simulink model "Unipolar_Carrier_Signal_Based_SVPWM"  (R2023a)
settings: Solver=VariableStepAuto  StartTime=0.0  StopTime=2  MaxStep=1e-5  RelTol=1e-3
libraries: spsMosfetLib x12, spsDiodeLib x6, simulink x4, spsVoltageMeasurementLib x4, spsDCVoltageSourceLib x2, spsGroundLib x2, spsSeriesRLCBranchLib x2, spsAsynchronousMachineSIUnitsLib x1, spsCurrentMeasurementLib x1, spsStairGeneratorLib x1, spsThreePhaseVIMeasurementLib x1, spspowerguiLib x1
settings Model: Creator=Vigneshwaran R  LastModifiedBy=Vigneshwaran R
settings DataIOCC: SaveOutput=off  SaveState=on  SignalLogging=off  DSMLogging=off  ReturnWorkspaceOutputs=off  LoggingToFile=on
settings ModelReferenceCC: EnableRefExpFcnMdlSchedulingChecks=on

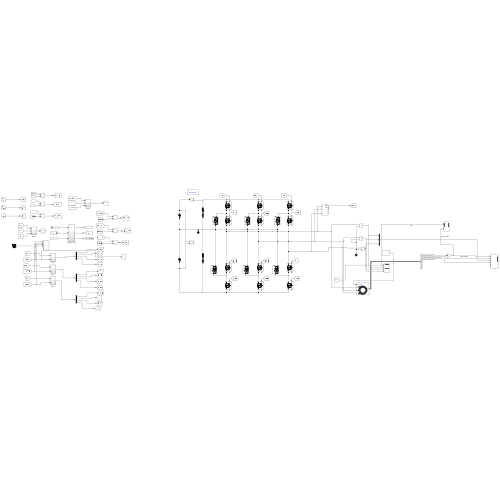
[thumbnail: Simulink's stored preview of the top-level diagram]
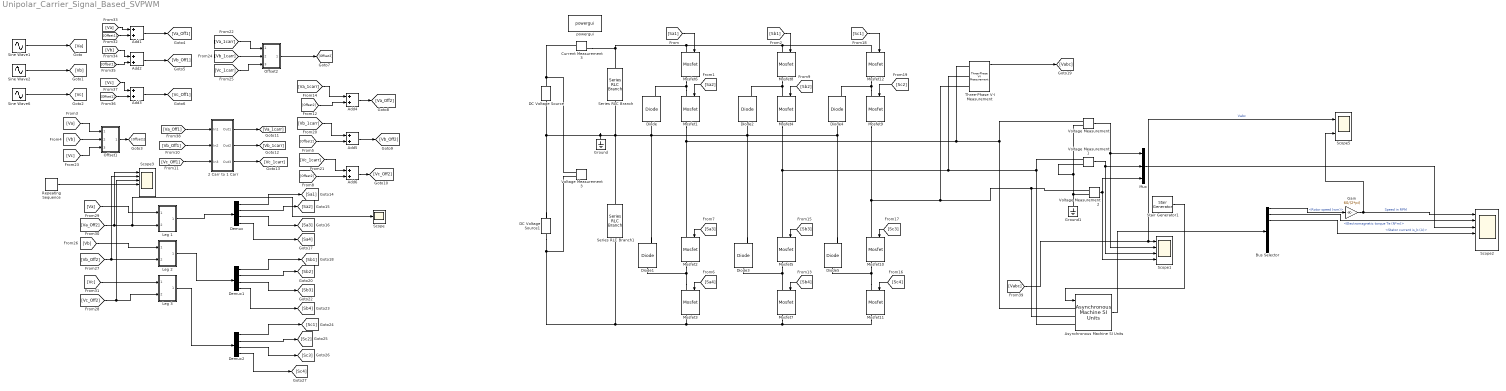
== system Unipolar_Carrier_Signal_Based_SVPWM ==
  2 Carr to 1 Carr : Subsystem
  Add{1..6} (6 alike) : Sum
  Asynchronous Machine SI Units : spsAsynchronousMachineSIUnitsLib/Asynchronous Machine SI Units  RotorType=Squirrel-cage  PresetModel="15:  5.4 HP (4KW)   400 V  50Hz 1430 RPM"  MechanicalLoad=Torque Tm  ShowDetailedParameters=on  ReferenceFrame=Rotor  Units=SI  MeasurementBus=off  NominalParameters=[4000 400 50]  VoltageRatio=1  Stator=[1.405 0.005839]  Rotor=[1.395 0.005839]  Cage1=[0.4155 0.002066]  Cage2=[0.4168 0.0003495]  Lm=0.1722  Mechanical=[0.0131 0.002985 2]  PolePairs=2  InitialConditions=[0 0 0 0 0 0 0 0]  SimulateSaturation=off  Saturation=[14.03593122, 27.81365428, 53.79336849, 72.68890987, 97.98006896, 148.6815601, 215.7428561, 302.9841135, 428.7778367 ; 230, 322, 414, 460, 506, 552, 598, 644, 690]  LoadFlowParameters=1492000  TsPowergui=0  TsBlock=-1  IterativeModel=Trapezoidal non iterative  IterativeDiscreteModel=Trapezoidal non iterative  Pmec=1.492e+006
  Bus Selector : BusSelector  OutputSignals=Mechanical.Rotor speed (wm),Mechanical.Electromagnetic torque Te (N*m),Stator measurements.Stator current is_b (A),Stator measurements.Stator flux phis_d (V s),Stator measurements.Stator flux phis_q (V s),Stator measurements.Stator current is_a (A),Stator measurements.Stator current is_b (A),Stator measurements.Stator current is_c (A)
  Current Measurement3 : spsCurrentMeasurementLib/Current Measurement  PhasorSimulation=off  OutputType=Complex  PSBequivalent=0
  DC Voltage Source : spsDCVoltageSourceLib/DC Voltage Source  Amplitude=380  Measurements=None
  DC Voltage Source1 : spsDCVoltageSourceLib/DC Voltage Source  Amplitude=380  Measurements=None
  Demux : Demux
  Demux1 : Demux
  Demux2 : Demux
  Diode{,1..5} (6 alike) : spsDiodeLib/Diode  Ron=0.001  Lon=0  Vf=0.8  IC=0  UseSnubber=0  Rs=500  Cs=250e-9  Measurements=on
  Gain : Gain  Gain=60/(2*pi)
  Ground : spsGroundLib/Ground  LConnTagsString=a
  Ground1 : spsGroundLib/Ground  LConnTagsString=a
  Leg 1 : Subsystem
  Leg 2 : Subsystem
  Leg 3 : Subsystem
  Mosfet{1..12} (12 alike) : spsMosfetLib/Mosfet  Ron=0.1  Lon=0  Rd=0.01  Vfd=0  IC=0  Rs=1e5  Cs=inf  Measurements=on
  Mux : Mux  Inputs=3
  Offset1 : Subsystem
  Offset2 : Subsystem
  Repeating Sequence : simulink/Sources/Repeating Sequence  rep_seq_t=[0 2.5e-5 5e-5 7.5e-5 10e-5]  rep_seq_y=[0.5 1 0.5 0 0.5 ]
  Scope : Scope
  Scope1 : Scope  NumInputPorts=4
  Scope2 : Scope  NumInputPorts=6
  Scope3 : Scope  NumInputPorts=6
  Scope5 : Scope  NumInputPorts=2
  Series RLC Branch : spsSeriesRLCBranchLib/Series RLC Branch  LConnTagsString=__new0  RConnTagsString=__new0  BranchType=RC  Resistance=0.1  Inductance=1e-3  SetiL0=off  InitialCurrent=0  Capacitance=4.7e-3  Setx0=off  InitialVoltage=0  Measurements=None
  Series RLC Branch1 : spsSeriesRLCBranchLib/Series RLC Branch  LConnTagsString=__new0  RConnTagsString=__new0  BranchType=RC  Resistance=0.1  Inductance=1e-3  SetiL0=off  InitialCurrent=0  Capacitance=4.7e-3  Setx0=off  InitialVoltage=0  Measurements=None
  Sine Wave1 : Sin  Frequency=2*pi*50  SampleTime=0
  Sine Wave2 : Sin  Frequency=2*pi*50  Phase=2*pi/3  SampleTime=0
  Sine Wave6 : Sin  Frequency=2*pi*50  Phase=4*pi/3  SampleTime=0
  Stair Generator1 : spsStairGeneratorLib/Stair Generator  t=[0 1]  e=[0 10]  Ts=0
  Three-Phase V-I Measurement : spsThreePhaseVIMeasurementLib/Three-Phase V-I Measurement  VoltageMeasurement=phase-to-phase  SetLabelV=off  LabelV=Vabc  Vpu=off  VpuLL=off  CurrentMeasurement=yes  SetLabelI=off  LabelI=Iabc  Ipu=off  Pbase=100e6  Vbase=500e3  OutputType=Complex  PhasorSimulation=off  PSBequivalent=0
  Voltage Measurement{,1..3} (4 alike) : spsVoltageMeasurementLib/Voltage Measurement  PhasorSimulation=off  OutputType=Complex  PSBequivalent=0
  powergui : spspowerguiLib/powergui  Priority=1  SimulationMode=Continuous  SampleTime=50e-6  frequency=60  Iterations=50  frequencyindice=50  Pbase=100e6  ErrMax=1e-4  UnitsV=kV  UnitsW=MW  buscounter=0  FunctionMessages=off  echomessages=off  EnableUseOfTLC=off  CurrentSourceSwitches=off  DisableSnubberDevices=off  DisableRonSwitches=off  DisableVfSwitches=off  DisplayEquations=off  AutomaticDiscreteSolvers=off  SolverType=Tustin/Backward Euler (TBE)  Interpol=off  ExternalGateDelay=off  methode=off  Ts=100  x0status=blocks  SPID=on  SwTol=0  HookPort=off  NonlinearTolerance=1e-4  nMaxIteration=100  ContinueOnMaxIteration=off  RestoreLinks=warning  ResistiveCurrentMeasurement=off  Frange=[0:2:500]  Ylog=off  Xlog=on  ShowGrid=off  save=off  variable=ZData  structure=0  ZoomFFT=off  StartTime=0.0  cycles=1  DisplayStyle=1  fundamental=60  FreqAxis=off  MaxFrequency=1000  frequencyindicesteady=1  RmsSteady=1  display=off
  wires:
  [Sa2] -> Mosfet1/1
  [Sa4] -> Mosfet3/1
  [Sa3] -> Mosfet2/1
  [Sa1] -> Mosfet6/1
  [Sb1] -> Mosfet8/1
  [Sb3] -> Mosfet5/1
  [Sb4] -> Mosfet7/1
  [Sb2] -> Mosfet4/1
  [Sc2] -> Mosfet9/1
  [Sc4] -> Mosfet11/1
  [Sc3] -> Mosfet10/1
  [Sc1] -> Mosfet12/1
  Three-Phase V-I Measurement/1 -> [Vabc]
  [Offset2] -> Add4/2
  [Va_1carr] -> Offset2/1(In1)
  [Offset2] -> Add5/2
  [Offset2] -> Add6/2
  [Vc] -> Leg 3/1(In1)
  [Va_1carr] -> Add4/1
  [Vb_1carr] -> Add5/1
  [Vb] -> Leg 2/1(In1)
  [Va] -> Leg 1/1(In1)
  [Vc_Off2] -> Leg 3/2(In2), Scope3/3
  Add6/1 -> [Vc_Off2]
  Add4/1 -> [Va_Off2]
  2 Carr to 1 Carr/3(Out3) -> [Vc_1carr]
  Offset2/1(Out1) -> [Offset2]
  [Vc_Off1] -> 2 Carr to 1 Carr/3(In3)
  2 Carr to 1 Carr/1(Out1) -> [Va_1carr]
  Offset1/1(Out1) -> [Offset1]
  [Vc_1carr] -> Offset2/3(In3)
  Add1/1 -> [Va_Off1]
  [Va] -> Offset1/1(In1)
  [Vc] -> Offset1/3(In3)
  [Vb] -> Offset1/2(In2)
  [Va_Off2] -> Scope3/1, Scope/1, Leg 1/2(In2)
  [Offset1] -> Add2/2
  [Vb] -> Add2/1
  Add5/1 -> [Vb_Off2]
  [Vb_Off1] -> 2 Carr to 1 Carr/2(In2)
  [Vb_1carr] -> Offset2/2(In2)
  [Offset1] -> Add3/2
  [Vb_Off2] -> Scope3/2, Leg 2/2(In2)
  [Va] -> Add1/1
  [Offset1] -> Add1/2
  [Vc] -> Add3/1
  [Vc_1carr] -> Add6/1
  2 Carr to 1 Carr/2(Out2) -> [Vb_1carr]
  [Va_Off1] -> 2 Carr to 1 Carr/1(In1)
  Add2/1 -> [Vb_Off1]
  Add3/1 -> [Vc_Off1]
  Leg 1/1(Out1) -> Demux/1
  Demux/1 -> [Sa1]
  Demux/2 -> [Sa2]
  Demux/3 -> [Sa3]
  Demux/4 -> [Sa4]
  Demux1/4 -> [Sb4]
  Demux1/3 -> [Sb3]
  Demux1/2 -> [Sb2]
  Demux1/1 -> [Sb1]
  Leg 2/1(Out1) -> Demux1/1
  Leg 3/1(Out1) -> Demux2/1
  Demux2/1 -> [Sc1]
  Demux2/2 -> [Sc2]
  Demux2/3 -> [Sc3]
  Demux2/4 -> [Sc4]
  Voltage Measurement/1 -> Mux/1, Scope1/2
  Voltage Measurement1/1 -> Scope1/3, Mux/2
  Voltage Measurement2/1 -> Scope1/4, Mux/3
  Mux/1 -> Scope2/3
  Asynchronous Machine SI Units/1 -> Bus Selector/1
  Bus Selector/1 -> Gain/1  "<Rotor speed (wm)>"
  Bus Selector/2 -> Scope2/2  "<Electromagnetic torque Te (N*m)>"
  Stair Generator1/1 -> Asynchronous Machine SI Units/1
  Repeating Sequence/1 -> Scope3/4
  Gain/1 -> Scope2/1, Scope5/2  "Speed in RPM"
  [Vabc] -> Scope5/1, Scope1/1  "Vabc"
  Bus Selector/3 -> Scope2/4  "<Stator current is_b (A)>"
  Sine Wave2/1 -> [Vb]
  Sine Wave1/1 -> [Va]
  Sine Wave6/1 -> [Vc]
  connections:
  Diode4/LConn1 -- Series RLC Branch1/LConn1 -- Series RLC Branch/RConn1 -- Ground/LConn1 -- DC Voltage Source/LConn1 -- DC Voltage Source1/RConn1 -- Diode1/RConn1 -- Diode/LConn1 -- Diode2/LConn1 -- Diode3/RConn1 -- Diode5/RConn1
  Series RLC Branch/LConn1 -- Current Measurement3/RConn1 -- Mosfet8/LConn1 -- Mosfet12/LConn1 -- Mosfet6/LConn1
  Mosfet3/LConn1 -- Mosfet2/RConn1 -- Diode1/LConn1
  Three-Phase V-I Measurement/LConn1 -- Mosfet1/RConn1 -- Mosfet2/LConn1 -- Asynchronous Machine SI Units/LConn1 -- Voltage Measurement/LConn1
  Mosfet1/LConn1 -- Mosfet6/RConn1 -- Diode/RConn1
  Voltage Measurement3/LConn2 -- DC Voltage Source1/LConn1 -- Series RLC Branch1/RConn1 -- Mosfet7/RConn1 -- Mosfet11/RConn1 -- Mosfet3/RConn1
  Mosfet5/RConn1 -- Mosfet7/LConn1 -- Diode3/LConn1
  Mosfet8/RConn1 -- Mosfet4/LConn1 -- Diode2/RConn1
  Mosfet11/LConn1 -- Mosfet10/RConn1 -- Diode5/LConn1
  Mosfet9/LConn1 -- Mosfet12/RConn1 -- Diode4/RConn1
  Mosfet4/RConn1 -- Asynchronous Machine SI Units/LConn3 -- Voltage Measurement1/LConn1 -- Three-Phase V-I Measurement/LConn2 -- Mosfet5/LConn1
  Mosfet9/RConn1 -- Asynchronous Machine SI Units/LConn2 -- Voltage Measurement2/LConn1 -- Three-Phase V-I Measurement/LConn3 -- Mosfet10/LConn1
  Current Measurement3/LConn1 -- Voltage Measurement3/LConn1 -- DC Voltage Source/RConn1
  Voltage Measurement/LConn2 -- Ground1/LConn1 -- Voltage Measurement2/LConn2 -- Voltage Measurement1/LConn2

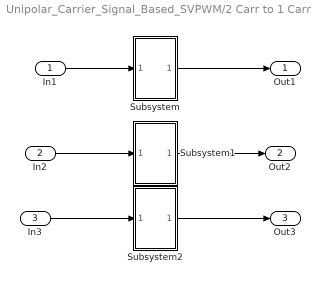
== system Unipolar_Carrier_Signal_Based_SVPWM/2 Carr to 1 Carr ==
  In1 : Inport
  In2 : Inport  Port=2
  In3 : Inport  Port=3
  Subsystem : Subsystem
  Subsystem1 : Subsystem
  Subsystem2 : Subsystem
  Out1 : Outport
  Out2 : Outport  Port=2
  Out3 : Outport  Port=3
  wires:
  In2/1 -> Subsystem1/1(In1)
  In3/1 -> Subsystem2/1(In1)
  Subsystem1/1(Out1) -> Out2/1
  Subsystem2/1(Out1) -> Out3/1
  Subsystem/1(Out1) -> Out1/1
  In1/1 -> Subsystem/1(In1)

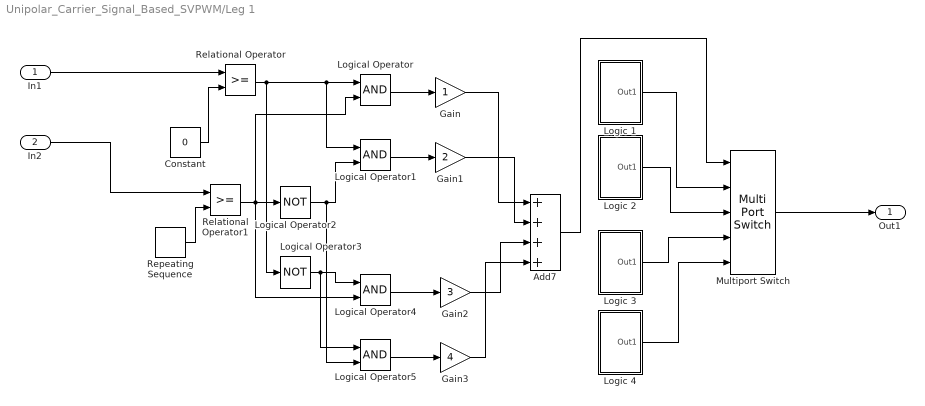
== system Unipolar_Carrier_Signal_Based_SVPWM/Leg 1 ==
  In1 : Inport
  In2 : Inport  Port=2
  Add7 : Sum  Inputs=++++
  Constant : Constant  Value=0
  Gain : Gain
  Gain1 : Gain  Gain=2
  Gain2 : Gain  Gain=3
  Gain3 : Gain  Gain=4
  Logic 1 : Subsystem
  Logic 2 : Subsystem
  Logic 3 : Subsystem
  Logic 4 : Subsystem
  Logical Operator{,1,4..5} (4 alike) : Logic  AllPortsSameDT=off  OutDataTypeStr=boolean
  Logical Operator2 : Logic  Operator=NOT  AllPortsSameDT=off  OutDataTypeStr=boolean
  Logical Operator3 : Logic  Operator=NOT  AllPortsSameDT=off  OutDataTypeStr=boolean
  Multiport Switch : MultiPortSwitch  Inputs=4  SaturateOnIntegerOverflow=off  InputSameDT=off
  Relational Operator : RelationalOperator  OutDataTypeStr=boolean  RndMeth=Simplest  InputSameDT=off
  Relational Operator1 : RelationalOperator  OutDataTypeStr=boolean  RndMeth=Simplest  InputSameDT=off
  Repeating Sequence : simulink/Sources/Repeating Sequence  rep_seq_t=[0 2.5e-5 5e-5 7.5e-5 10e-5]  rep_seq_y=[0.5 1 0.5 0 0.5 ]
  Out1 : Outport
  wires:
  Logical Operator5/1 -> Gain3/1
  Logical Operator1/1 -> Gain1/1
  Constant/1 -> Relational Operator/2
  Logical Operator3/1 -> Logical Operator5/1, Logical Operator4/1
  Logic 4/1(Out1) -> Multiport Switch/5
  Logical Operator4/1 -> Gain2/1
  Logical Operator2/1 -> Logical Operator5/2, Logical Operator1/2
  Relational Operator1/1 -> Logical Operator4/2, Logical Operator2/1, Logical Operator/2
  Gain2/1 -> Add7/3
  In2/1 -> Relational Operator1/1
  Add7/1 -> Multiport Switch/1
  Repeating Sequence/1 -> Relational Operator1/2
  Relational Operator/1 -> Logical Operator3/1, Logical Operator1/1, Logical Operator/1
  Logic 3/1(Out1) -> Multiport Switch/4
  Gain/1 -> Add7/1
  Gain1/1 -> Add7/2
  Logic 2/1(Out1) -> Multiport Switch/3
  Logic 1/1(Out1) -> Multiport Switch/2
  Gain3/1 -> Add7/4
  Logical Operator/1 -> Gain/1
  Multiport Switch/1 -> Out1/1
  In1/1 -> Relational Operator/1

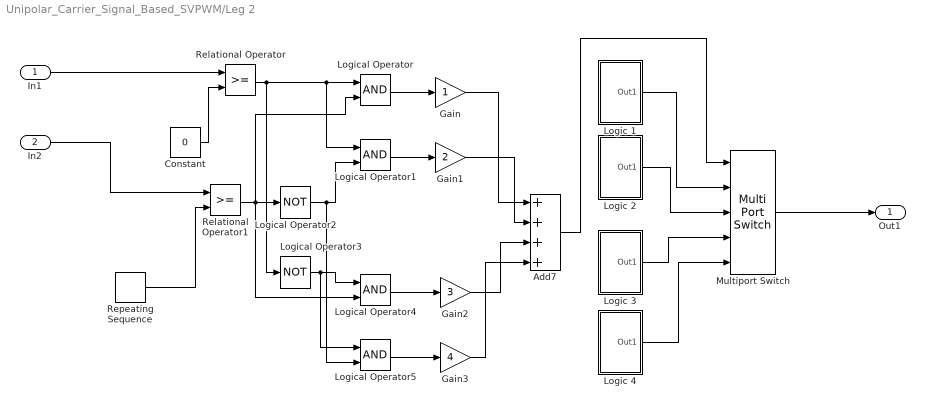
== system Unipolar_Carrier_Signal_Based_SVPWM/Leg 2 ==
  In1 : Inport
  In2 : Inport  Port=2
  Add7 : Sum  Inputs=++++
  Constant : Constant  Value=0
  Gain : Gain
  Gain1 : Gain  Gain=2
  Gain2 : Gain  Gain=3
  Gain3 : Gain  Gain=4
  Logic 1 : Subsystem
  Logic 2 : Subsystem
  Logic 3 : Subsystem
  Logic 4 : Subsystem
  Logical Operator{,1,4..5} (4 alike) : Logic  AllPortsSameDT=off  OutDataTypeStr=boolean
  Logical Operator2 : Logic  Operator=NOT  AllPortsSameDT=off  OutDataTypeStr=boolean
  Logical Operator3 : Logic  Operator=NOT  AllPortsSameDT=off  OutDataTypeStr=boolean
  Multiport Switch : MultiPortSwitch  Inputs=4  SaturateOnIntegerOverflow=off  InputSameDT=off
  Relational Operator : RelationalOperator  OutDataTypeStr=boolean  RndMeth=Simplest  InputSameDT=off
  Relational Operator1 : RelationalOperator  OutDataTypeStr=boolean  RndMeth=Simplest  InputSameDT=off
  Repeating Sequence : simulink/Sources/Repeating Sequence  rep_seq_t=[0 2.5e-5 5e-5 7.5e-5 10e-5]  rep_seq_y=[0.5 1 0.5 0 0.5 ]
  Out1 : Outport
  wires:
  In1/1 -> Relational Operator/1
  Multiport Switch/1 -> Out1/1
  Logical Operator/1 -> Gain/1
  Gain3/1 -> Add7/4
  Logic 1/1(Out1) -> Multiport Switch/2
  Logic 2/1(Out1) -> Multiport Switch/3
  Gain1/1 -> Add7/2
  Gain/1 -> Add7/1
  Logic 3/1(Out1) -> Multiport Switch/4
  Relational Operator/1 -> Logical Operator/1, Logical Operator1/1, Logical Operator3/1
  Repeating Sequence/1 -> Relational Operator1/2
  Add7/1 -> Multiport Switch/1
  In2/1 -> Relational Operator1/1
  Gain2/1 -> Add7/3
  Relational Operator1/1 -> Logical Operator/2, Logical Operator2/1, Logical Operator4/2
  Logical Operator2/1 -> Logical Operator1/2, Logical Operator5/2
  Logical Operator4/1 -> Gain2/1
  Logic 4/1(Out1) -> Multiport Switch/5
  Logical Operator3/1 -> Logical Operator4/1, Logical Operator5/1
  Constant/1 -> Relational Operator/2
  Logical Operator1/1 -> Gain1/1
  Logical Operator5/1 -> Gain3/1

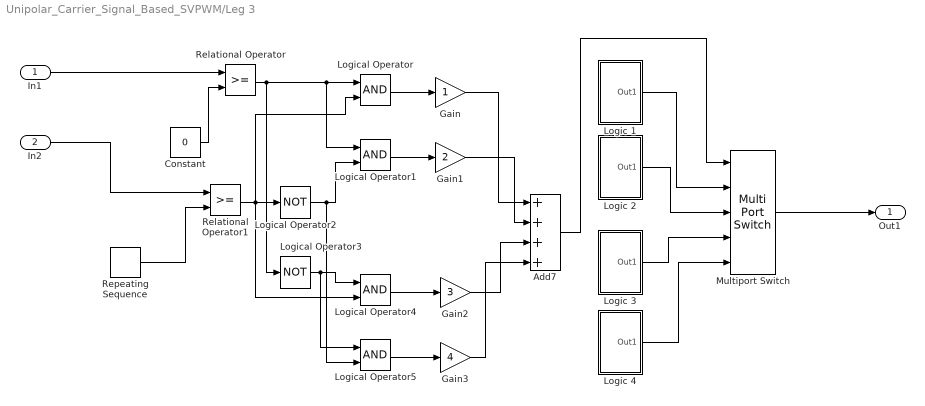
== system Unipolar_Carrier_Signal_Based_SVPWM/Leg 3 ==
  In1 : Inport
  In2 : Inport  Port=2
  Add7 : Sum  Inputs=++++
  Constant : Constant  Value=0
  Gain : Gain
  Gain1 : Gain  Gain=2
  Gain2 : Gain  Gain=3
  Gain3 : Gain  Gain=4
  Logic 1 : Subsystem
  Logic 2 : Subsystem
  Logic 3 : Subsystem
  Logic 4 : Subsystem
  Logical Operator{,1,4..5} (4 alike) : Logic  AllPortsSameDT=off  OutDataTypeStr=boolean
  Logical Operator2 : Logic  Operator=NOT  AllPortsSameDT=off  OutDataTypeStr=boolean
  Logical Operator3 : Logic  Operator=NOT  AllPortsSameDT=off  OutDataTypeStr=boolean
  Multiport Switch : MultiPortSwitch  Inputs=4  SaturateOnIntegerOverflow=off  InputSameDT=off
  Relational Operator : RelationalOperator  OutDataTypeStr=boolean  RndMeth=Simplest  InputSameDT=off
  Relational Operator1 : RelationalOperator  OutDataTypeStr=boolean  RndMeth=Simplest  InputSameDT=off
  Repeating Sequence : simulink/Sources/Repeating Sequence  rep_seq_t=[0 2.5e-5 5e-5 7.5e-5 10e-5]  rep_seq_y=[0.5 1 0.5 0 0.5 ]
  Out1 : Outport
  wires:
  Logical Operator5/1 -> Gain3/1
  Logical Operator1/1 -> Gain1/1
  Constant/1 -> Relational Operator/2
  Logical Operator3/1 -> Logical Operator5/1, Logical Operator4/1
  Logic 4/1(Out1) -> Multiport Switch/5
  Logical Operator4/1 -> Gain2/1
  Logical Operator2/1 -> Logical Operator5/2, Logical Operator1/2
  Relational Operator1/1 -> Logical Operator4/2, Logical Operator2/1, Logical Operator/2
  Gain2/1 -> Add7/3
  In2/1 -> Relational Operator1/1
  Add7/1 -> Multiport Switch/1
  Repeating Sequence/1 -> Relational Operator1/2
  Relational Operator/1 -> Logical Operator3/1, Logical Operator1/1, Logical Operator/1
  Logic 3/1(Out1) -> Multiport Switch/4
  Gain/1 -> Add7/1
  Gain1/1 -> Add7/2
  Logic 2/1(Out1) -> Multiport Switch/3
  Logic 1/1(Out1) -> Multiport Switch/2
  Gain3/1 -> Add7/4
  Logical Operator/1 -> Gain/1
  Multiport Switch/1 -> Out1/1
  In1/1 -> Relational Operator/1

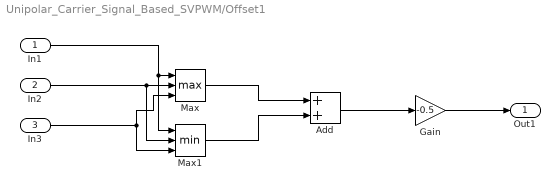
== system Unipolar_Carrier_Signal_Based_SVPWM/Offset1 ==
  In1 : Inport
  In2 : Inport  Port=2
  In3 : Inport  Port=3
  Add : Sum
  Gain : Gain  Gain=-0.5
  Max : MinMax  Function=max  Inputs=3
  Max1 : MinMax  Inputs=3
  Out1 : Outport
  wires:
  In2/1 -> Max1/2, Max/2
  In1/1 -> Max1/1, Max/1
  Max/1 -> Add/1
  In3/1 -> Max/3, Max1/3
  Gain/1 -> Out1/1
  Max1/1 -> Add/2
  Add/1 -> Gain/1

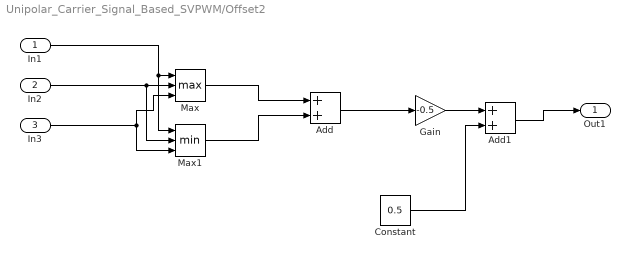
== system Unipolar_Carrier_Signal_Based_SVPWM/Offset2 ==
  In1 : Inport
  In2 : Inport  Port=2
  In3 : Inport  Port=3
  Add : Sum
  Add1 : Sum
  Constant : Constant  Value=0.5
  Gain : Gain  Gain=-0.5
  Max : MinMax  Function=max  Inputs=3
  Max1 : MinMax  Inputs=3
  Out1 : Outport
  wires:
  Add/1 -> Gain/1
  Max1/1 -> Add/2
  In3/1 -> Max1/3, Max/3
  Max/1 -> Add/1
  In1/1 -> Max/1, Max1/1
  In2/1 -> Max/2, Max1/2
  Gain/1 -> Add1/1
  Constant/1 -> Add1/2
  Add1/1 -> Out1/1

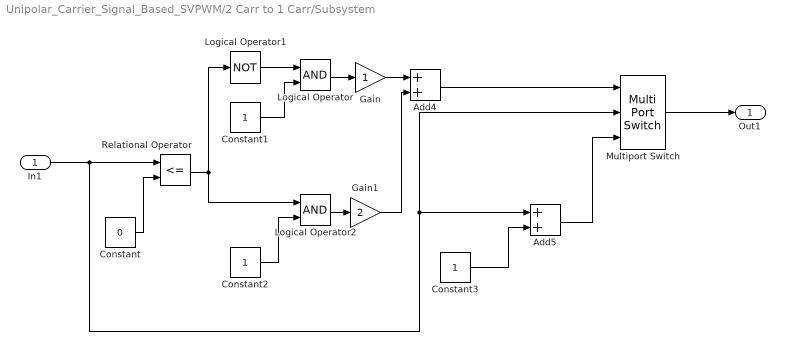
== system Unipolar_Carrier_Signal_Based_SVPWM/2 Carr to 1 Carr/Subsystem ==
  In1 : Inport
  Add4 : Sum
  Add5 : Sum
  Constant : Constant  Value=0
  Constant1 : Constant
  Constant2 : Constant
  Constant3 : Constant
  Gain : Gain
  Gain1 : Gain  Gain=2
  Logical Operator : Logic  AllPortsSameDT=off  OutDataTypeStr=boolean
  Logical Operator1 : Logic  Operator=NOT  AllPortsSameDT=off  OutDataTypeStr=boolean
  Logical Operator2 : Logic  AllPortsSameDT=off  OutDataTypeStr=boolean
  Multiport Switch : MultiPortSwitch  Inputs=2  SaturateOnIntegerOverflow=off  InputSameDT=off
  Relational Operator : RelationalOperator  Operator=<=  OutDataTypeStr=boolean  RndMeth=Simplest  InputSameDT=off
  Out1 : Outport
  wires:
  Gain1/1 -> Add4/2
  In1/1 -> Relational Operator/1, Add5/1, Multiport Switch/2
  Add5/1 -> Multiport Switch/3
  Logical Operator1/1 -> Logical Operator/1
  Logical Operator/1 -> Gain/1
  Constant1/1 -> Logical Operator/2
  Logical Operator2/1 -> Gain1/1
  Multiport Switch/1 -> Out1/1
  Gain/1 -> Add4/1
  Relational Operator/1 -> Logical Operator1/1, Logical Operator2/1
  Constant2/1 -> Logical Operator2/2
  Constant/1 -> Relational Operator/2
  Add4/1 -> Multiport Switch/1
  Constant3/1 -> Add5/2

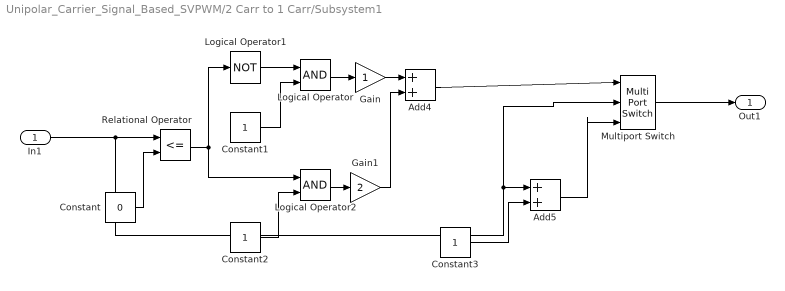
== system Unipolar_Carrier_Signal_Based_SVPWM/2 Carr to 1 Carr/Subsystem1 ==
  In1 : Inport
  Add4 : Sum
  Add5 : Sum
  Constant : Constant  Value=0
  Constant1 : Constant
  Constant2 : Constant
  Constant3 : Constant
  Gain : Gain
  Gain1 : Gain  Gain=2
  Logical Operator : Logic  AllPortsSameDT=off  OutDataTypeStr=boolean
  Logical Operator1 : Logic  Operator=NOT  AllPortsSameDT=off  OutDataTypeStr=boolean
  Logical Operator2 : Logic  AllPortsSameDT=off  OutDataTypeStr=boolean
  Multiport Switch : MultiPortSwitch  Inputs=2  SaturateOnIntegerOverflow=off  InputSameDT=off
  Relational Operator : RelationalOperator  Operator=<=  OutDataTypeStr=boolean  RndMeth=Simplest  InputSameDT=off
  Out1 : Outport
  wires:
  Constant3/1 -> Add5/2
  Add4/1 -> Multiport Switch/1
  Constant/1 -> Relational Operator/2
  Constant2/1 -> Logical Operator2/2
  Relational Operator/1 -> Logical Operator2/1, Logical Operator1/1
  Gain/1 -> Add4/1
  Multiport Switch/1 -> Out1/1
  Logical Operator2/1 -> Gain1/1
  Constant1/1 -> Logical Operator/2
  Logical Operator/1 -> Gain/1
  Logical Operator1/1 -> Logical Operator/1
  Add5/1 -> Multiport Switch/3
  In1/1 -> Relational Operator/1, Add5/1, Multiport Switch/2
  Gain1/1 -> Add4/2

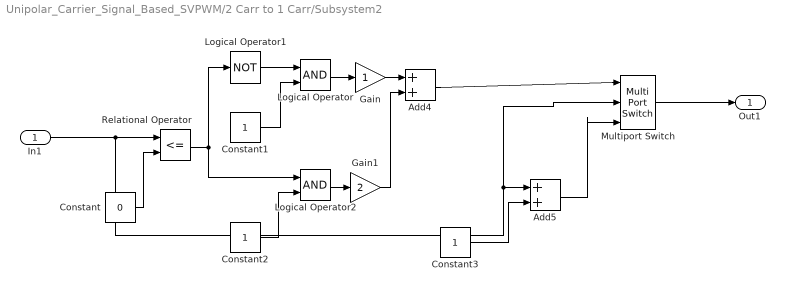
== system Unipolar_Carrier_Signal_Based_SVPWM/2 Carr to 1 Carr/Subsystem2 ==
  In1 : Inport
  Add4 : Sum
  Add5 : Sum
  Constant : Constant  Value=0
  Constant1 : Constant
  Constant2 : Constant
  Constant3 : Constant
  Gain : Gain
  Gain1 : Gain  Gain=2
  Logical Operator : Logic  AllPortsSameDT=off  OutDataTypeStr=boolean
  Logical Operator1 : Logic  Operator=NOT  AllPortsSameDT=off  OutDataTypeStr=boolean
  Logical Operator2 : Logic  AllPortsSameDT=off  OutDataTypeStr=boolean
  Multiport Switch : MultiPortSwitch  Inputs=2  SaturateOnIntegerOverflow=off  InputSameDT=off
  Relational Operator : RelationalOperator  Operator=<=  OutDataTypeStr=boolean  RndMeth=Simplest  InputSameDT=off
  Out1 : Outport
  wires:
  Gain1/1 -> Add4/2
  In1/1 -> Multiport Switch/2, Add5/1, Relational Operator/1
  Add5/1 -> Multiport Switch/3
  Logical Operator1/1 -> Logical Operator/1
  Logical Operator/1 -> Gain/1
  Constant1/1 -> Logical Operator/2
  Logical Operator2/1 -> Gain1/1
  Multiport Switch/1 -> Out1/1
  Gain/1 -> Add4/1
  Relational Operator/1 -> Logical Operator1/1, Logical Operator2/1
  Constant2/1 -> Logical Operator2/2
  Constant/1 -> Relational Operator/2
  Add4/1 -> Multiport Switch/1
  Constant3/1 -> Add5/2

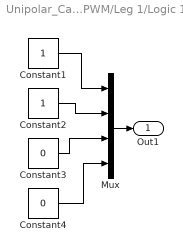
== system Unipolar_Carrier_Signal_Based_SVPWM/Leg 1/Logic 1 ==
  Constant1 : Constant
  Constant2 : Constant
  Constant3 : Constant  Value=0
  Constant4 : Constant  Value=0
  Mux : Mux
  Out1 : Outport
  wires:
  Constant1/1 -> Mux/1
  Constant2/1 -> Mux/2
  Mux/1 -> Out1/1
  Constant4/1 -> Mux/4
  Constant3/1 -> Mux/3

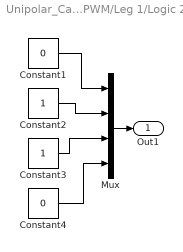
== system Unipolar_Carrier_Signal_Based_SVPWM/Leg 1/Logic 2 ==
  Constant1 : Constant  Value=0
  Constant2 : Constant
  Constant3 : Constant
  Constant4 : Constant  Value=0
  Mux : Mux
  Out1 : Outport
  wires:
  Constant3/1 -> Mux/3
  Constant4/1 -> Mux/4
  Mux/1 -> Out1/1
  Constant2/1 -> Mux/2
  Constant1/1 -> Mux/1

== system Unipolar_Carrier_Signal_Based_SVPWM/Leg 1/Logic 3 ==
  Constant1 : Constant  Value=0
  Constant2 : Constant
  Constant3 : Constant
  Constant4 : Constant  Value=0
  Mux : Mux
  Out1 : Outport
  wires:
  Constant1/1 -> Mux/1
  Constant2/1 -> Mux/2
  Mux/1 -> Out1/1
  Constant4/1 -> Mux/4
  Constant3/1 -> Mux/3

== system Unipolar_Carrier_Signal_Based_SVPWM/Leg 1/Logic 4 ==
  Constant1 : Constant  Value=0
  Constant2 : Constant  Value=0
  Constant3 : Constant
  Constant4 : Constant
  Mux : Mux
  Out1 : Outport
  wires:
  Constant3/1 -> Mux/3
  Constant4/1 -> Mux/4
  Mux/1 -> Out1/1
  Constant2/1 -> Mux/2
  Constant1/1 -> Mux/1

== system Unipolar_Carrier_Signal_Based_SVPWM/Leg 2/Logic 1 ==
  Constant1 : Constant
  Constant2 : Constant
  Constant3 : Constant  Value=0
  Constant4 : Constant  Value=0
  Mux : Mux
  Out1 : Outport
  wires:
  Constant3/1 -> Mux/3
  Constant4/1 -> Mux/4
  Mux/1 -> Out1/1
  Constant2/1 -> Mux/2
  Constant1/1 -> Mux/1

== system Unipolar_Carrier_Signal_Based_SVPWM/Leg 2/Logic 2 ==
  Constant1 : Constant  Value=0
  Constant2 : Constant
  Constant3 : Constant
  Constant4 : Constant  Value=0
  Mux : Mux
  Out1 : Outport
  wires:
  Constant1/1 -> Mux/1
  Constant2/1 -> Mux/2
  Mux/1 -> Out1/1
  Constant4/1 -> Mux/4
  Constant3/1 -> Mux/3

== system Unipolar_Carrier_Signal_Based_SVPWM/Leg 2/Logic 3 ==
  Constant1 : Constant  Value=0
  Constant2 : Constant
  Constant3 : Constant
  Constant4 : Constant  Value=0
  Mux : Mux
  Out1 : Outport
  wires:
  Constant3/1 -> Mux/3
  Constant4/1 -> Mux/4
  Mux/1 -> Out1/1
  Constant2/1 -> Mux/2
  Constant1/1 -> Mux/1

== system Unipolar_Carrier_Signal_Based_SVPWM/Leg 2/Logic 4 ==
  Constant1 : Constant  Value=0
  Constant2 : Constant  Value=0
  Constant3 : Constant
  Constant4 : Constant
  Mux : Mux
  Out1 : Outport
  wires:
  Constant1/1 -> Mux/1
  Constant2/1 -> Mux/2
  Mux/1 -> Out1/1
  Constant4/1 -> Mux/4
  Constant3/1 -> Mux/3

== system Unipolar_Carrier_Signal_Based_SVPWM/Leg 3/Logic 1 ==
  Constant1 : Constant
  Constant2 : Constant
  Constant3 : Constant  Value=0
  Constant4 : Constant  Value=0
  Mux : Mux
  Out1 : Outport
  wires:
  Constant1/1 -> Mux/1
  Constant2/1 -> Mux/2
  Mux/1 -> Out1/1
  Constant4/1 -> Mux/4
  Constant3/1 -> Mux/3

== system Unipolar_Carrier_Signal_Based_SVPWM/Leg 3/Logic 2 ==
  Constant1 : Constant  Value=0
  Constant2 : Constant
  Constant3 : Constant
  Constant4 : Constant  Value=0
  Mux : Mux
  Out1 : Outport
  wires:
  Constant3/1 -> Mux/3
  Constant4/1 -> Mux/4
  Mux/1 -> Out1/1
  Constant2/1 -> Mux/2
  Constant1/1 -> Mux/1

== system Unipolar_Carrier_Signal_Based_SVPWM/Leg 3/Logic 3 ==
  Constant1 : Constant  Value=0
  Constant2 : Constant
  Constant3 : Constant
  Constant4 : Constant  Value=0
  Mux : Mux
  Out1 : Outport
  wires:
  Constant1/1 -> Mux/1
  Constant2/1 -> Mux/2
  Mux/1 -> Out1/1
  Constant4/1 -> Mux/4
  Constant3/1 -> Mux/3

== system Unipolar_Carrier_Signal_Based_SVPWM/Leg 3/Logic 4 ==
  Constant1 : Constant  Value=0
  Constant2 : Constant  Value=0
  Constant3 : Constant
  Constant4 : Constant
  Mux : Mux
  Out1 : Outport
  wires:
  Constant3/1 -> Mux/3
  Constant4/1 -> Mux/4
  Mux/1 -> Out1/1
  Constant2/1 -> Mux/2
  Constant1/1 -> Mux/1
